simulink model "TCM_controls"  (Simulink 8.1)
settings: Solver=ode45  StartTime=0.0  StopTime=10.0  RelTol=1e-3
undefined symbols (not defined in the file): bias, sgn, sigbuilder_block, sldvsubsys, StatesInp
libraries: simulink x4, sldvlib x1
(part 1 of 2)
settings Model: Creator=mddavies  LastModifiedBy=mddavies
settings DataIOCC: SignalLoggingSaveFormat=Dataset
settings OptimizationCC: ExpressionDepthLimit=128
settings DebuggingCC: FcnCallInpInsideContextMsg=EnableAllAsError
settings GRTTargetCC: CombineOutputUpdateFcns=on  GRTInterface=off

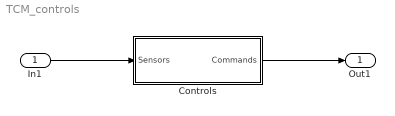
== system TCM_controls ==
  In1 : Inport
  Controls : Subsystem  RequirementInfo={} %GIDa_bfda8087_8264_4058_aa1c_dac31995074c
  Out1 : Outport
  wires:
  Controls/1(Commands) -> Out1/1
  In1/1 -> Controls/1(Sensors)

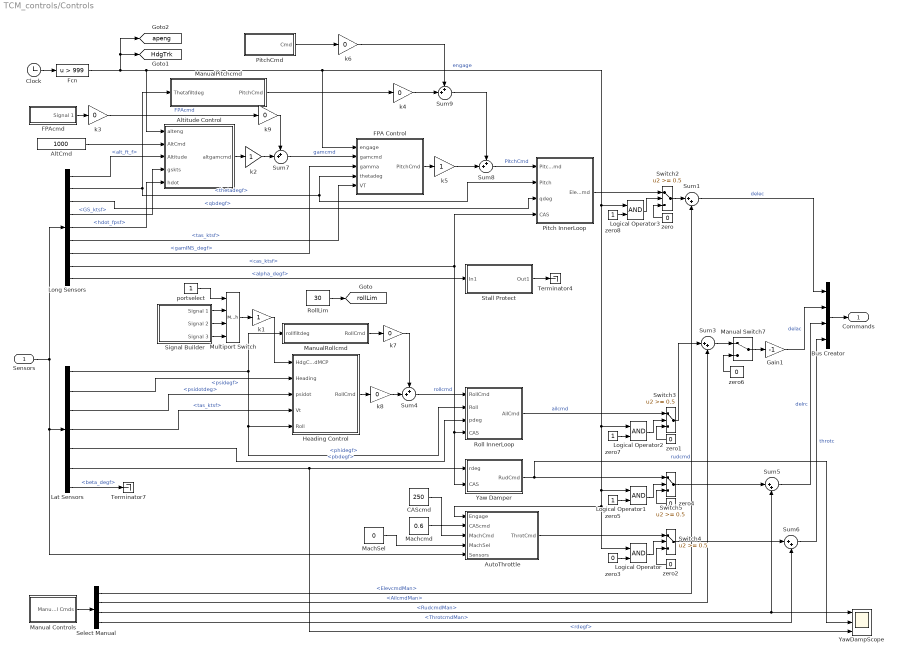
== system TCM_controls/Controls ==
  Sensors : Inport  RequirementInfo={} %GIDa_70f77869_2cec_4ef4_8031_6b1ced368b4e
  AltCmd : Constant  RequirementInfo={} %GIDa_dec5e6b5_3f45_4fcc_9d07_233f77b9af99  Value=1000
  Altitude Control : Subsystem  RequirementInfo={'other' '..\..\tcm_requirements.docx' '@Simulink_requirement_item_14' 'true' 'Altitude Control' '' } %GIDa_c6f0573f_5709_411f_9273_5bd8edb6dccb
  AutoThrottle : Subsystem  RequirementInfo={'other' '..\..\tcm_requirements.docx' '@Simulink_requirement_item_20' 'true' 'Auto Throttle' '' } %GIDa_acd8b2ec_afb4_4e6d_93a7_fadc15d05afd
  Bus Creator : BusCreator  RequirementInfo={} %GIDa_98b05b2e_4f50_4eac_8142_7ba35f876d49
  CAScmd : Constant  RequirementInfo={} %GIDa_a292a332_f5c6_4f14_a0b0_05556e3e387a  Value=250
  Clock : Clock
      settings: RequirementInfo={} %GIDa_53558b21_c326_4915_aa80_3e38ab183ff3
  FPA Control : Subsystem  RequirementInfo={'other' '..\..\tcm_requirements.docx' '@Simulink_requirement_item_15' 'true' 'FPA Control' '' } %GIDa_dac5565b_9328_42f5_a37f_49e511e4f966
  FPAcmd : Subsystem  Tag=STV Subsys  RequirementInfo={} %GIDa_1bafd98b_d710_4002_989e_dd755c1a6c5b  LoadFcn=sigbuilder_block('load');  StartFcn=sigbuilder_block('start');  StopFcn=sigbuilder_block('stop');  ClipboardFcn=sigbuilder_block('clipboard');  mask(Sigbuilder block){}
      mask help: Sigbuilder GUI
      mask init:
      | if ~strcmp(get_param(bdroot(gcbh),'SimulationStatus'),'stopped') tuvar = sigbuilder_block('maskInit'); end
      settings: CopyFcn=sigbuilder_block('copy');  DeleteFcn=sigbuilder_block('delete');  ModelCloseFcn=sigbuilder_block('modelClose');  PreSaveFcn=sigbuilder_block('preSave');  PauseFcn=sigbuilder_block('pause')  ContinueFcn=sigbuilder_block('continue')  NameChangeFcn=sigbuilder_block('namechange');  OpenFcn=sigbuilder_block('open',[437.6 199.2 550.4 400 ]);  CloseFcn=sigbuilder_block('close');
      mask Display: plot(0,0,100,100,[10,10,40,40,10],[80,20,20,80,80],[40,10],[50,50], [40,27,10],[65,72,56],[40,25,25,10],[28,28,43,43]);
  Fcn : Fcn  RequirementInfo={} %GIDa_18158dea_7053_4aed_9677_b2431daf36da  Expr=u > 999
  Gain1 : Gain  RequirementInfo={} %GIDa_de67ea91_cef0_4311_be02_dc516f1dcbf6  Gain=-1  SaturateOnIntegerOverflow=on  OutDataTypeStr=Inherit: Same as input  ParamDataTypeStr=Inherit: Same as input
  Heading Control : Subsystem  RequirementInfo={'other' '..\..\tcm_requirements.docx' '@Simulink_requirement_item_16' 'true' 'Heading Control' '' } %GIDa_4d0d22af_8d69_4b73_8cc8_bf810aba30d0
  Lat Sensors : BusSelector  RequirementInfo={} %GIDa_bff82875_4bac_4e5e_ab39_128c86e45cef  OutputSignals=phidegf,psidegf,EulerRates.psidotdeg,tas_ktsf,pbdegf,rdegf,beta_degf
  Logical Operator : Logic  RequirementInfo={} %GIDa_c9271ae6_5d7e_4e57_a9b4_c4e93f533c75  AllPortsSameDT=off  OutDataTypeStr=boolean
  Logical Operator1 : Logic  RequirementInfo={} %GIDa_bf47c128_6073_4620_9be0_bb5310186e50  AllPortsSameDT=off  OutDataTypeStr=boolean
  Logical Operator2 : Logic  RequirementInfo={} %GIDa_16878af7_9208_4803_a632_79b1d2b562ea  AllPortsSameDT=off  OutDataTypeStr=boolean
  Logical Operator3 : Logic  RequirementInfo={} %GIDa_ac9639de_92a9_41be_9497_96302f0b2ccb  AllPortsSameDT=off  OutDataTypeStr=boolean
  Long Sensors : BusSelector  RequirementInfo={} %GIDa_05f26765_1655_42bc_bb4b_9210360e7e03  OutputSignals=alt_ft_f,thetadegf,qbdegf,GS_ktsf,hdot_fpsf,tas_ktsf,gamINS_degf,cas_ktsf,alpha_degf
  MachSel : Constant  RequirementInfo={} %GIDa_406d0f5f_5220_4552_95b2_2b4717a09293  Value=0
  Machcmd : Constant  RequirementInfo={} %GIDa_bb2c15e6_ad11_44f7_ab52_0e2f70039c12  Value=0.6
  Manual Controls : Subsystem  RequirementInfo={} %GIDa_f3a5a448_da82_4163_b7bb_5bb62cb3bee1
  Manual Switch7 : ManualSwitch  RequirementInfo={} %GIDa_238d4b35_b042_4032_9af2_039cd16e9328
  ManualPitchcmd : Subsystem  RequirementInfo={} %GIDa_6f844cf0_ae74_4e05_a5ad_b4b8e37a6781
  ManualRollcmd : Subsystem  RequirementInfo={} %GIDa_c6f4980f_561d_4e8c_856f_74806f1ad0aa
  Multiport Switch : MultiPortSwitch  RequirementInfo={} %GIDa_7f9fa05b_ab44_4b7a_9c8e_e05a1b0a73ae
  Pitch InnerLoop : Subsystem  RequirementInfo={'other' '..\..\tcm_requirements.docx' '@Simulink_requirement_item_17' 'true' 'Pitch InnerLoop' '' } %GIDa_4ed92d47_0400_4ecc_8db1_4e64c2e8d840
  PitchCmd : Subsystem  RequirementInfo={} %GIDa_d85db5dc_c2d2_453e_abb8_0bd5f726e4bb
  Roll InnerLoop : Subsystem  RequirementInfo={'other' '..\..\tcm_requirements.docx' '@Simulink_requirement_item_18' 'true' 'Roll InnerLoop' '' } %GIDa_823e046a_cfe1_4d55_9112_ea4cd7fe46ad
  RollLim : Constant  RequirementInfo={} %GIDa_230728ed_bde8_446c_b764_b18561e20cc4  Value=30
  Select Manual : BusSelector  RequirementInfo={} %GIDa_92fe7b47_3580_4d0c_9647_4bc53b6f9b8a  OutputSignals=ElevcmdMan,AilcmdMan,RudcmdMan,ThrotcmdMan
  Signal Builder : Subsystem  Tag=STV Subsys  RequirementInfo={} %GIDa_de104f81_7e09_48dc_b266_08630f3c268d  LoadFcn=sigbuilder_block('load');  StartFcn=sigbuilder_block('start');  StopFcn=sigbuilder_block('stop');  ClipboardFcn=sigbuilder_block('clipboard');  mask(Sigbuilder block){}
      mask help: Sigbuilder GUI
      mask init:
      | if ~strcmp(get_param(bdroot(gcbh),'SimulationStatus'),'stopped') tuvar = sigbuilder_block('maskInit'); end
      settings: CopyFcn=sigbuilder_block('copy');  DeleteFcn=sigbuilder_block('delete');  ModelCloseFcn=sigbuilder_block('modelClose');  PreSaveFcn=sigbuilder_block('preSave');  PauseFcn=sigbuilder_block('pause')  ContinueFcn=sigbuilder_block('continue')  NameChangeFcn=sigbuilder_block('namechange');  OpenFcn=sigbuilder_block('open',[436.656 200.842 549.567 399.685 ]);  CloseFcn=sigbuilder_block('close');
      mask Display: plot(0,0,100,100,[10,10,40,40,10],[80,20,20,80,80],[40,10],[50,50], [40,27,10],[65,72,56],[40,25,25,10],[28,28,43,43]);
  Stall Protect : Subsystem  RequirementInfo={} %GIDa_81308623_113c_47aa_8ecf_809416eeaa1d
  Sum1 : Sum  RequirementInfo={} %GIDa_93388a83_d69c_4626_a784_0212b19640c2  Inputs=|++
  Sum3 : Sum  RequirementInfo={} %GIDa_5b146ea8_0844_4ecc_b2ed_46e902b595f5  Inputs=|++
  Sum4 : Sum  RequirementInfo={} %GIDa_f08d028e_f47a_4873_80ef_83f18a12d8bd  Inputs=++|
  Sum5 : Sum  RequirementInfo={} %GIDa_31e1df87_937a_4eae_9557_7a21f34925e9  Inputs=|++
  Sum6 : Sum  RequirementInfo={} %GIDa_d2e78c48_42e1_4808_ae96_99a07762e7f0  Inputs=|++
  Sum7 : Sum  RequirementInfo={} %GIDa_e99670bf_988f_4456_ae22_5591ba30988f  Inputs=++|
  Sum8 : Sum  RequirementInfo={} %GIDa_3a0866c5_ad06_43cb_b2cc_1f5b5b613d25  Inputs=++|
  Sum9 : Sum  RequirementInfo={} %GIDa_154a2fe3_c154_42b0_99bf_ba40407caa09  Inputs=++|
  Switch2 : Switch  RequirementInfo={} %GIDa_d498c400_8384_4eff_abe5_abc2c2cb970a  Threshold=0.5
  Switch3 : Switch  RequirementInfo={} %GIDa_3149d6ff_f1dc_4a93_8707_7aaa0bfbdbc5  Threshold=0.5
  Switch4 : Switch  RequirementInfo={} %GIDa_474c7c0a_d693_431e_8c01_caaa5ad223f0  Threshold=0.5
  Switch5 : Switch  RequirementInfo={} %GIDa_12969d2f_7aeb_457e_8b61_46499c9d1588  Threshold=0.5
  Terminator4 : Terminator
      settings: RequirementInfo={} %GIDa_d981aeba_8485_4cf6_9549_0eb875528307
  Terminator7 : Terminator
      settings: RequirementInfo={} %GIDa_903322f5_1a87_4f88_820f_b96602a5e0f1
  Yaw Damper : Subsystem  RequirementInfo={'other' '..\..\tcm_requirements.docx' '@Simulink_requirement_item_19' 'true' 'Yaw Damper' '' } %GIDa_e03d9e3b_12d1_4127_985c_f09d6aa1a0d4
  YawDampScope : Scope  NumInputPorts=3
      settings: RequirementInfo={} %GIDa_6e94e61d_629b_4b33_92c3_ceaeeee69283  YMin=-5~-5~-5  YMax=5~5~5  SaveName=ScopeData4
  k1 : Gain  RequirementInfo={} %GIDa_b8ae6e56_e541_4fc9_8c33_5b640a1878bf
  k2 : Gain  RequirementInfo={} %GIDa_6764272f_c68a_4a56_bdfa_0b378ddcd164
  k3 : Gain  RequirementInfo={} %GIDa_36ed0483_434a_4689_a994_f7e4d4d3ba8b  Gain=0
  k4 : Gain  RequirementInfo={} %GIDa_b90d9015_94ab_49f8_a57e_54f0da0033c5  Gain=0
  k5 : Gain  RequirementInfo={} %GIDa_6d0bd2a3_b291_46d0_acba_fbe7503f71f4
  k6 : Gain  RequirementInfo={} %GIDa_6ec47e81_80e4_46c7_bb08_7322656805f5  Gain=0
  k7 : Gain  RequirementInfo={} %GIDa_df4ad79b_1a76_4940_a29a_64f1606d84a6  Gain=0
  k8 : Gain  RequirementInfo={} %GIDa_1da1ea53_366f_4084_b3ea_cbc5e4466241  Gain=0
  k9 : Gain  RequirementInfo={} %GIDa_927c2f41_014f_4868_b1e4_5880ae857acb  Gain=0
  portselect : Constant  RequirementInfo={} %GIDa_8a2376e2_46a6_49b2_81f8_f473a2c2615b
  zero : Constant  RequirementInfo={} %GIDa_8a55f2a8_d8df_42ae_895a_6e79a0ece0e3  Value=0
  zero1 : Constant  RequirementInfo={} %GIDa_c41a1b2d_1ac1_4b5c_8545_bea2e4ad18df  Value=0
  zero2 : Constant  RequirementInfo={} %GIDa_ba22c0b1_8245_4fd4_a8d4_a7971c18af40  Value=0
  zero3 : Constant  RequirementInfo={} %GIDa_f2feaf15_c205_4351_8c8b_f665221607f7  Value=0
  zero4 : Constant  RequirementInfo={} %GIDa_7305b391_df8e_4170_9236_a6d6d9a3b599  Value=0
  zero5 : Constant  RequirementInfo={} %GIDa_c492baed_9fe4_4b04_ac61_664bb274daf7
  zero6 : Constant  RequirementInfo={} %GIDa_337c7813_2094_4eef_ae7b_8f96373121b3  Value=0
  zero7 : Constant  RequirementInfo={} %GIDa_6f701eca_c5af_4506_bbf1_05e4ee92343b
  zero8 : Constant  RequirementInfo={} %GIDa_681bde8a_1fca_46f3_8a9f_42ee6d0a1930
  Commands : Outport  RequirementInfo={} %GIDa_935988b2_9427_4adc_b718_1a527609e997
  tag scope: HdgTrk=global, apeng=global, rollLim=global
  wires:
  Lat Sensors/6 -> YawDampScope/3, Yaw Damper/1(rdeg)  "<rdegf>"
  Lat Sensors/5 -> Roll InnerLoop/3(pdeg)  "<pbdegf>"
  Lat Sensors/4 -> Heading Control/4(Vt)  "<tas_ktsf>"
  Lat Sensors/3 -> Heading Control/3(psidot)  "<psidotdeg>"
  Lat Sensors/2 -> Heading Control/2(Heading)  "<psidegf>"
  Lat Sensors/1 -> Heading Control/5(Roll), Roll InnerLoop/2(Roll), ManualRollcmd/1(rollfiltdeg)  "<phidegf>"
  AutoThrottle/1(ThrotCmd) -> Switch4/1
  Sum6/1 -> Bus Creator/4  "throtc"
  Sum5/1 -> Bus Creator/3  "delrc"
  Gain1/1 -> Bus Creator/2  "delac"
  Sum1/1 -> Bus Creator/1  "delec"
  Bus Creator/1 -> Commands/1
  Manual Switch7/1 -> Gain1/1
  k9/1 -> Sum7/1
  k3/1 -> k9/1  "FPAcmd"
  k2/1 -> Sum7/2
  Sensors/1 -> Long Sensors/1, Lat Sensors/1, AutoThrottle/5(Sensors)
  Long Sensors/1 -> Altitude Control/3(Altitude)  "<alt_ft_f>"
  Long Sensors/2 -> Pitch InnerLoop/2(Pitch), FPA Control/4(thetadeg), ManualPitchcmd/1(Thetafiltdeg)  "<thetadegf>"
  Long Sensors/8 -> Roll InnerLoop/4(CAS), Yaw Damper/2(CAS), Pitch InnerLoop/4(CAS)  "<cas_ktsf>"
  Long Sensors/7 -> FPA Control/3(gamma)  "<gamINS_degf>"
  Long Sensors/9 -> Stall Protect/1(In1)  "<alpha_degf>"
  Clock/1 -> Fcn/1
  Manual Controls/1(Manual Cmds) -> Select Manual/1
  Select Manual/1 -> Sum1/2  "<ElevcmdMan>"
  Lat Sensors/7 -> Terminator7/1  "<beta_degf>"
  Sum3/1 -> Manual Switch7/1
  Select Manual/2 -> Sum3/2  "<AilcmdMan>"
  Switch3/1 -> Sum3/1
  Sum4/1 -> Roll InnerLoop/1(RollCmd)  "rollcmd"
  Switch5/1 -> Sum5/1
  Select Manual/3 -> Sum5/2, YawDampScope/1  "<RudcmdMan>"
  CAScmd/1 -> AutoThrottle/2(CAScmd)
  Switch4/1 -> Sum6/1
  Select Manual/4 -> Sum6/2  "<ThrotcmdMan>"
  AltCmd/1 -> Altitude Control/2(AltCmd)
  k8/1 -> Sum4/2
  zero6/1 -> Manual Switch7/2
  ManualRollcmd/1(RollCmd) -> k7/1
  Switch2/1 -> Sum1/1
  zero/1 -> Switch2/3
  Fcn/1 -> Altitude Control/1(alteng), FPA Control/1(engage), Logical Operator3/1, Logical Operator2/1, Logical Operator1/1, Logical Operator/1, AutoThrottle/1(Engage), [apeng], [HdgTrk]  "engage"
  Pitch InnerLoop/1(ElevCmd) -> Switch2/1
  Altitude Control/1(altgamcmd) -> k2/1
  Sum8/1 -> Pitch InnerLoop/1(PitchCmd)  "PitchCmd"
  ManualPitchcmd/1(PitchCmd) -> k4/1
  k5/1 -> Sum8/2
  FPA Control/1(PitchCmd) -> k5/1
  Long Sensors/5 -> Altitude Control/5(hdot)  "<hdot_fpsf>"
  Sum7/1 -> FPA Control/2(gamcmd)  "gamcmd"
  Heading Control/1(RollCmd) -> k8/1
  zero1/1 -> Switch3/3
  Roll InnerLoop/1(AilCmd) -> Switch3/1  "ailcmd"
  Logical Operator/1 -> Switch4/2
  zero3/1 -> Logical Operator/2
  zero4/1 -> Switch5/3
  Logical Operator1/1 -> Switch5/2
  zero5/1 -> Logical Operator1/2
  Yaw Damper/1(RudCmd) -> Switch5/1, YawDampScope/2  "rudcmd"
  zero7/1 -> Logical Operator2/2
  Logical Operator2/1 -> Switch3/2
  zero8/1 -> Logical Operator3/2
  Logical Operator3/1 -> Switch2/2
  FPAcmd/1(Signal 1) -> k3/1
  k7/1 -> Sum4/1
  portselect/1 -> Multiport Switch/1
  Signal Builder/1(Signal 1) -> Multiport Switch/2
  Signal Builder/2(Signal 2) -> Multiport Switch/3
  Signal Builder/3(Signal 3) -> Multiport Switch/4
  Multiport Switch/1 -> k1/1
  RollLim/1 -> [rollLim]
  k1/1 -> Heading Control/1(HdgCmdMCP)
  Stall Protect/1(Out1) -> Terminator4/1
  k4/1 -> Sum9/2
  PitchCmd/1(Cmd) -> k6/1
  Sum9/1 -> Sum8/1
  k6/1 -> Sum9/1
  Long Sensors/3 -> Pitch InnerLoop/3(qdeg)  "<qbdegf>"
  Long Sensors/4 -> Altitude Control/4(gskts)  "<GS_ktsf>"
  Long Sensors/6 -> FPA Control/5(VT)  "<tas_ktsf>"
  Machcmd/1 -> AutoThrottle/3(MachCmd)
  MachSel/1 -> AutoThrottle/4(MachSel)
  zero2/1 -> Switch4/3

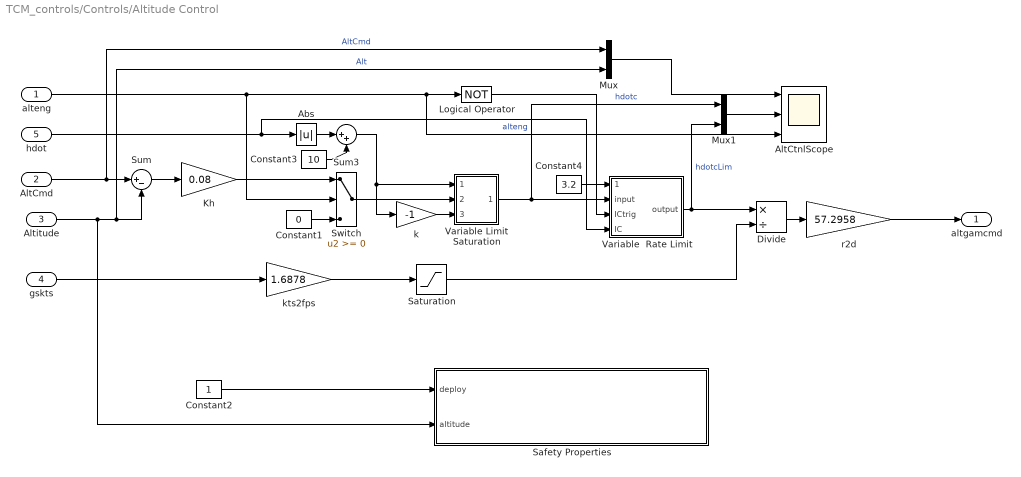
== system TCM_controls/Controls/Altitude Control ==
  alteng : Inport  RequirementInfo={} %GIDa_02633e80_0791_4996_845b_8463c8d13bdc
  AltCmd : Inport  RequirementInfo={} %GIDa_f01a5c64_5048_4ead_817f_1150ce5bafcd  Port=2
  Altitude : Inport  RequirementInfo={} %GIDa_53c75335_2a6f_43ef_8904_84222eeb9f50  Port=3
  gskts : Inport  RequirementInfo={} %GIDa_c10c2a4f_902c_4e8b_96b8_b4689bb09c59  Port=4
  hdot : Inport  RequirementInfo={} %GIDa_f0efc3ce_aa23_4913_b248_8bb3483f1443  Port=5
  Abs : Abs  RequirementInfo={} %GIDa_584ef2d4_6be5_48a2_82b7_54540d88e5ea  SaturateOnIntegerOverflow=on
  AltCtnlScope : Scope  NumInputPorts=3
      settings: RequirementInfo={} %GIDa_d2af245a_14d1_44a1_b76f_5993cea8ac6e  TimeRange=30  YMin=10000~-5~0  YMax=10200~15~1  SaveName=ScopeData3
  Constant1 : Constant  RequirementInfo={} %GIDa_142be318_071c_4741_b70e_6146455c6752  Value=0
  Constant2 : Constant  RequirementInfo={} %GIDa_aee2841a_d62a_4778_8195_69efdbd9f66c
  Constant3 : Constant  RequirementInfo={} %GIDa_4fd9daa6_86dd_480b_9e87_d7cd7d3e5ab7  Value=10
  Constant4 : Constant  RequirementInfo={} %GIDa_7712bef4_2805_4e51_9a6e_1aedf3857e74  Value=3.2
  Divide : Product  RequirementInfo={} %GIDa_518615b6_8a21_4c19_89cc_0075a8168445  Inputs=*/
  Kh : Gain  RequirementInfo={} %GIDa_2ef3e796_3e8a_4861_921e_724dc1fdaaf3  Gain=0.08
  Logical Operator : Logic  RequirementInfo={} %GIDa_dfcb40e8_cce6_4bbe_8389_8e071fcd808f  Operator=NOT
  Mux : Mux  RequirementInfo={} %GIDa_4ebb49f9_be23_440d_8228_36b8343cd879  Inputs=2
  Mux1 : Mux  RequirementInfo={} %GIDa_24366faa_de64_4cd5_a201_bde413c56619  Inputs=2
  Safety Properties : Subsystem  Tag=VerificationSubsystem  RequirementInfo={} %GIDa_fe9274ab_2722_4454_bf71_2814ec7d0b9e  DisableCoverage=on  LoadFcn=sldvsubsys('check')  TreatAsAtomicUnit=on  SimViewingDevice=on  mask(VerificationSubsystem){}
      mask init:
      | sldvsubsys('maskInit');
      settings: CopyFcn=sldvsubsys('copy');  OpenFcn=open_system(gcb,'force');
      settings: PreSaveFcn=|
      | set_param(gcb,'SimViewingDevice','on');
      | sldvsubsys('check');
      mask Help: helpview(fullfile(docroot,'toolbox','sldv','sldv.map'),'verificationsubsystem')
      mask Display: image(imread('sldvicon_versubsys.png','BackGroundColor',[1 1 1]),'center');
  Saturation : Saturate  RequirementInfo={} %GIDa_286fe06e_20c7_4df1_a50b_74f682ccfd1b  UpperLimit=1000  LowerLimit=0.0001
  Sum : Sum  RequirementInfo={} %GIDa_6fe83580_1e8a_49e8_b370_a5304e817a17  Inputs=|+-
  Sum3 : Sum  RequirementInfo={} %GIDa_2bc31f57_20de_45df_96a4_7a5cdc2ac6df  Inputs=|++  SaturateOnIntegerOverflow=on  InputSameDT=on  OutDataTypeStr=Inherit: Same as first input
  Switch : Switch  RequirementInfo={} %GIDa_d475166c_c2c0_4927_9fa4_f3e5ea7f613c
  Variable  Rate Limit : Subsystem  RequirementInfo={} %GIDa_e32f4459_34b6_4548_91a5_a7d4babef003
  Variable Limit Saturation : Subsystem  RequirementInfo={} %GIDa_15178d5d_84e2_4ba5_8f7e_4b2d48b0fa42
  k : Gain  RequirementInfo={} %GIDa_fef99285_5710_42fb_a83f_a209dfb615da  Gain=-1
  kts2fps : Gain  RequirementInfo={} %GIDa_ea7b234f_3d40_4e67_9a2d_14996b1d35d3  Gain=1.6878
  r2d : Gain  RequirementInfo={} %GIDa_7936e5b9_2b56_40ef_b6e3_68e6a59e37bd  Gain=57.2958
  altgamcmd : Outport  RequirementInfo={} %GIDa_75dd3768_76b3_4bf1_aedb_56b7c675b7de
  wires:
  Sum/1 -> Kh/1
  AltCmd/1 -> Sum/1, Mux/1  "AltCmd"
  Altitude/1 -> Safety Properties/2(altitude), Sum/2, Mux/2  "Alt"
  hdot/1 -> Abs/1, Variable  Rate Limit/4(IC)
  Abs/1 -> Sum3/1
  Constant3/1 -> Sum3/2
  k/1 -> Variable Limit Saturation/3(Lo_lim)
  Sum3/1 -> k/1, Variable Limit Saturation/1(up_lim)
  alteng/1 -> Switch/2, Logical Operator/1, AltCtnlScope/3  "alteng"
  gskts/1 -> kts2fps/1
  Divide/1 -> r2d/1
  r2d/1 -> altgamcmd/1
  Logical Operator/1 -> Variable  Rate Limit/3(ICtrig)
  Variable Limit Saturation/1(Out1) -> Variable  Rate Limit/2(input), Mux1/1  "hdotc"
  Constant4/1 -> Variable  Rate Limit/1(ratelim)
  Variable  Rate Limit/1(output) -> Divide/1, Mux1/2  "hdotcLim"
  kts2fps/1 -> Saturation/1
  Saturation/1 -> Divide/2
  Switch/1 -> Variable Limit Saturation/2(SigIn)
  Kh/1 -> Switch/1
  Constant1/1 -> Switch/3
  Mux/1 -> AltCtnlScope/1
  Mux1/1 -> AltCtnlScope/2
  Constant2/1 -> Safety Properties/1(deploy)

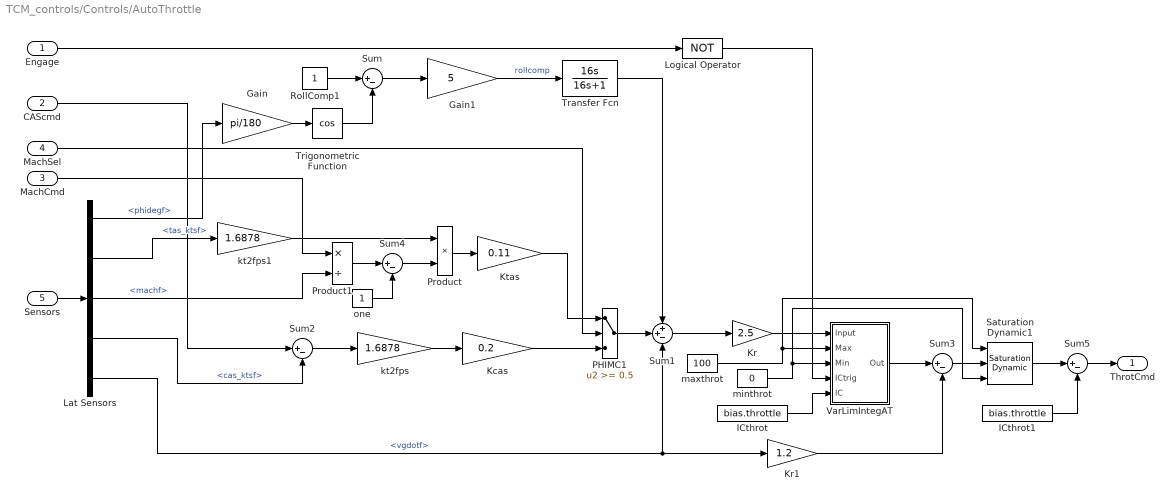
== system TCM_controls/Controls/AutoThrottle ==
  Engage : Inport  RequirementInfo={} %GIDa_c78350fb_fa81_4a6c_8041_709e76a511d5
  CAScmd : Inport  RequirementInfo={} %GIDa_d62d65f5_bfde_45ec_b3c2_4a1562c916d6  Port=2
  MachCmd : Inport  RequirementInfo={} %GIDa_6e18ebad_ed77_45d2_aa73_dcf4bccb826c  Port=3
  MachSel : Inport  RequirementInfo={} %GIDa_e1e0a91a_092e_4073_8070_c3a59f5b97f0  Port=4
  Sensors : Inport  RequirementInfo={} %GIDa_04629c4c_6ba1_49d3_8fc4_922875642bf0  Port=5
  Gain : Gain  RequirementInfo={} %GIDa_f72af6a8_661d_4465_a155_21ee211addf4  Gain=pi/180
  Gain1 : Gain  RequirementInfo={} %GIDa_d1c1e1b8_ce39_46fd_8f6a_f7539e22cf0a  Gain=5
  ICthrot : Constant  RequirementInfo={} %GIDa_2fcdee91_9306_45f9_9b2a_322564fd6a9a  Value=bias.throttle  SampleTime=-1
  ICthrot1 : Constant  RequirementInfo={} %GIDa_e3cb9808_12a0_449b_a4a7_26c21a0dd8b2  Value=bias.throttle  SampleTime=-1
  Kcas : Gain  RequirementInfo={} %GIDa_ac1acf1d_597b_4e61_a972_9454b39e0927  Gain=0.2
  Kr : Gain  RequirementInfo={} %GIDa_db49a02a_6b80_49c5_91c0_1fbc690ab318  Gain=2.5
  Kr1 : Gain  RequirementInfo={} %GIDa_73ff3e33_02cb_4dbd_abf2_ecfbb60a33a4  Gain=1.2
  Ktas : Gain  RequirementInfo={} %GIDa_3937ba58_9f30_4ce2_9403_44b9fbdbbcdb  Gain=0.11
  Lat Sensors : BusSelector  RequirementInfo={} %GIDa_d4684bc5_15b9_4aca_86c1_b91af86b245e  OutputSignals=phidegf,tas_ktsf,machf,cas_ktsf,vgdotf
  Logical Operator : Logic  RequirementInfo={} %GIDa_4512f38f_f881_42c2_9fc9_d7785cd1fe48  Operator=NOT  AllPortsSameDT=off  OutDataTypeStr=boolean
  PHIMC1 : Switch  RequirementInfo={} %GIDa_38937a7f_5f70_4f47_9d3f_4f45007894cb  Threshold=0.5  SampleTime=0.02  SaturateOnIntegerOverflow=on
  Product : Product  RequirementInfo={} %GIDa_9d6aee68_f232_4ee5_a7bb_5058db639735  RndMeth=Zero
  Product1 : Product  RequirementInfo={} %GIDa_9bd25c5e_ccc8_467b_beb1_404913d69c67  Inputs=*/  RndMeth=Zero
  RollComp1 : Constant  RequirementInfo={} %GIDa_6f64c878_e625_47af_bbbc_1f46b151678b  SampleTime=-1
  Saturation Dynamic1 : simulink/Discontinuities/Saturation Dynamic  RequirementInfo={} %GIDa_9fa3fc13_ab06_443e_852f_62ed3f5eb5ad  OutMin=[]  OutMax=[]  OutDataTypeStr=Inherit: Same as second input  OutDataType=sfix(16)  OutScaling=2^-10  DoSatur=off
  Sum : Sum  RequirementInfo={} %GIDa_c96b5531_0d8e_4ce9_972a_a12a3c140a36  Inputs=|+-
  Sum1 : Sum  RequirementInfo={} %GIDa_ff122384_47e7_4541_b600_e49509ecbdcb  Inputs=++-
  Sum2 : Sum  RequirementInfo={} %GIDa_2a4657ac_602b_42c1_9aef_62135f38a158  Inputs=|+-
  Sum3 : Sum  RequirementInfo={} %GIDa_b04521ce_5b21_43fe_adca_81cc300ef696  Inputs=|+-
  Sum4 : Sum  RequirementInfo={} %GIDa_66decbf6_63a3_4144_8b9d_0f9ac1e88bb6  Inputs=|+-
  Sum5 : Sum  RequirementInfo={} %GIDa_00c82fc8_7d29_4e94_bb47_a680e8082b0d  Inputs=|+-
  Transfer Fcn : TransferFcn  RequirementInfo={} %GIDa_8a88fa97_6339_4910_8a70_ee6567c6dac7  Numerator=[16 0]  Denominator=[16 1]
  Trigonometric Function : Trigonometry  RequirementInfo={} %GIDa_e383f247_a1b6_4070_acb4_f0617f4ed0f0  Operator=cos
  VarLimIntegAT : Subsystem  RequirementInfo={} %GIDa_f396fc90_a185_45e5_987a_0bb57ea297cb
  kt2fps : Gain  RequirementInfo={} %GIDa_1fc554ce_56ee_47bc_880a_0cca1ceec330  Gain=1.6878
  kt2fps1 : Gain  RequirementInfo={} %GIDa_7ac87cf0_6bf6_4d0a_a4bc_65e2bc24c465  Gain=1.6878
  maxthrot : Constant  RequirementInfo={} %GIDa_9fb28dbc_f107_4823_9058_9630c9255e8b  Value=100  SampleTime=-1
  minthrot : Constant  RequirementInfo={} %GIDa_c621bed3_d7f5_471f_a710_16dd9df2d68f  Value=0  SampleTime=-1
  one : Constant  RequirementInfo={} %GIDa_cd20c5fe_ca4b_4fec_b358_54a99c4323c8  SampleTime=-1
  ThrotCmd : Outport  RequirementInfo={} %GIDa_da1d0932_be70_457f_b044_35341889dcb0
  wires:
  CAScmd/1 -> Sum2/1
  Sum2/1 -> kt2fps/1
  Sum1/1 -> Kr/1
  kt2fps/1 -> Kcas/1
  Kr/1 -> VarLimIntegAT/1(Input)
  Lat Sensors/5 -> Sum1/3, Kr1/1  "<vgdotf>"
  Kr1/1 -> Sum3/2
  Gain1/1 -> Transfer Fcn/1  "rollcomp"
  Sum/1 -> Gain1/1
  Trigonometric Function/1 -> Sum/2
  RollComp1/1 -> Sum/1
  Gain/1 -> Trigonometric Function/1
  Product1/1 -> Sum4/1
  one/1 -> Sum4/2
  Sum4/1 -> Product/2
  kt2fps1/1 -> Product/1
  Product/1 -> Ktas/1
  ICthrot/1 -> VarLimIntegAT/5(IC)
  Sum5/1 -> ThrotCmd/1
  ICthrot1/1 -> Sum5/2
  maxthrot/1 -> VarLimIntegAT/2(Max), Saturation Dynamic1/1
  minthrot/1 -> VarLimIntegAT/3(Min), Saturation Dynamic1/3
  VarLimIntegAT/1(Out) -> Sum3/1
  Sum3/1 -> Saturation Dynamic1/2
  Saturation Dynamic1/1 -> Sum5/1
  PHIMC1/1 -> Sum1/2
  Kcas/1 -> PHIMC1/3
  Ktas/1 -> PHIMC1/1
  Transfer Fcn/1 -> Sum1/1
  Sensors/1 -> Lat Sensors/1
  Lat Sensors/1 -> Gain/1  "<phidegf>"
  Lat Sensors/2 -> kt2fps1/1  "<tas_ktsf>"
  Lat Sensors/4 -> Sum2/2  "<cas_ktsf>"
  Logical Operator/1 -> VarLimIntegAT/4(ICtrig)
  Engage/1 -> Logical Operator/1
  MachSel/1 -> PHIMC1/2
  MachCmd/1 -> Product1/1
  Lat Sensors/3 -> Product1/2  "<machf>"

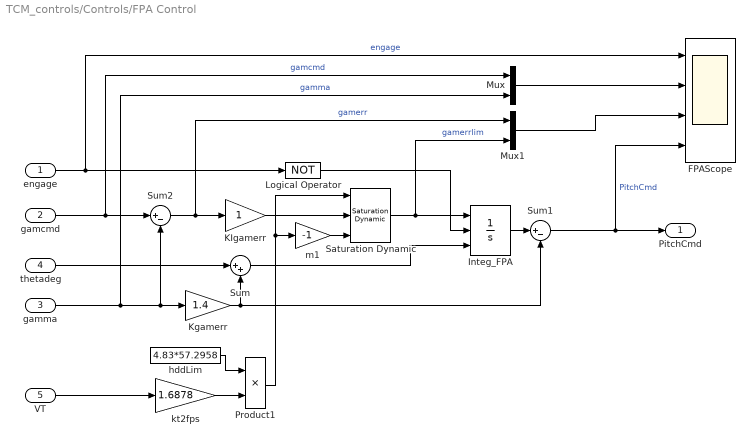
== system TCM_controls/Controls/FPA Control ==
  engage : Inport  RequirementInfo={} %GIDa_91c37145_4feb_4e56_8ba4_c1444bccd725
  gamcmd : Inport  RequirementInfo={} %GIDa_35b48e29_8b9c_4d71_bc7e_7f801982c35c  Port=2
  gamma : Inport  RequirementInfo={} %GIDa_7cbea00d_7d0f_450c_a5ed_a36a9e878ad0  Port=3
  thetadeg : Inport  RequirementInfo={} %GIDa_4586afe0_6b15_41e1_92d5_c5cb5fb147ef  Port=4
  VT : Inport  RequirementInfo={} %GIDa_6bfccaa8_1761_4626_8ec4_ffc0a99026f2  Port=5
  FPAScope : Scope  NumInputPorts=4
      settings: RequirementInfo={} %GIDa_6521d4bd_734b_43fe_9864_4305ee45935d  YMin=-1~-5~-2~-5  YMax=2~5~2~10  SaveName=ScopeData12
  Integ_FPA : Integrator  RequirementInfo={} %GIDa_4618b833_ba21_4a0d_a2fc_2134a3fdeaf2  ExternalReset=level  InitialConditionSource=external  IgnoreLimit=on
  KIgamerr : Gain  RequirementInfo={} %GIDa_e7aeae8d_827d_4b55_88b8_d1146319fac7
  Kgamerr : Gain  RequirementInfo={} %GIDa_86f0c6f9_3df3_4585_b0c9_834159dda395  Gain=1.4
  Logical Operator : Logic  RequirementInfo={} %GIDa_38a821e1_72c6_4a66_890a_b37f371667cc  Operator=NOT  AllPortsSameDT=off  OutDataTypeStr=boolean
  Mux : Mux  RequirementInfo={} %GIDa_00ae75ae_0d91_468f_8bef_95619be93ca4  Inputs=2
  Mux1 : Mux  RequirementInfo={} %GIDa_1f83504d_893a_4b09_bc5e_37512c768209  Inputs=2
  Product1 : Product  RequirementInfo={} %GIDa_6a4eb71a_e02e_42ca_b616_9047e49f49ad  RndMeth=Zero
  Saturation Dynamic : simulink/Discontinuities/Saturation Dynamic  RequirementInfo={} %GIDa_44aa7d72_cca6_47f1_9171_f5724db5be1d  OutMin=[]  OutMax=[]  OutDataTypeStr=Inherit: Same as second input  OutDataType=fixdt(1, 16)  OutScaling=2^-10  DoSatur=off
  Sum : Sum  RequirementInfo={} %GIDa_d76ccd44_16d8_45d1_a5c8_8cb855f3fa60  Inputs=|++
  Sum1 : Sum  RequirementInfo={} %GIDa_b2cc6a5b_6a0c_43d6_8e07_ed52d21ae106  Inputs=|+-
  Sum2 : Sum  RequirementInfo={} %GIDa_face43d4_08a8_46f4_83de_258637401c1a  Inputs=|+-
  hddLim : Constant  RequirementInfo={} %GIDa_33972148_d26a_40f1_920d_6c8d069e5033  Value=4.83*57.2958
  kt2fps : Gain  RequirementInfo={} %GIDa_000eb7a6_2566_45a9_a1f0_9c22b86ad75e  Gain=1.6878
  m1 : Gain  RequirementInfo={} %GIDa_5ffae559_17f0_4758_b2a4_292a59072b8b  Gain=-1
  PitchCmd : Outport  RequirementInfo={} %GIDa_d8cb079f_c0bb_4316_969b_9657e50c7147
  wires:
  Sum1/1 -> PitchCmd/1, FPAScope/4  "PitchCmd"
  Kgamerr/1 -> Sum1/2, Sum/2
  Integ_FPA/1 -> Sum1/1
  gamma/1 -> Kgamerr/1, Sum2/2, Mux/2  "gamma"
  thetadeg/1 -> Sum/1
  Sum/1 -> Integ_FPA/3
  engage/1 -> Logical Operator/1, FPAScope/1  "engage"
  Logical Operator/1 -> Integ_FPA/2
  kt2fps/1 -> Product1/2
  hddLim/1 -> Product1/1
  Product1/1 -> Saturation Dynamic/1, m1/1
  VT/1 -> kt2fps/1
  Saturation Dynamic/1 -> Integ_FPA/1, Mux1/2  "gamerrlim"
  KIgamerr/1 -> Saturation Dynamic/2
  m1/1 -> Saturation Dynamic/3
  Sum2/1 -> KIgamerr/1, Mux1/1  "gamerr"
  gamcmd/1 -> Sum2/1, Mux/1  "gamcmd"
  Mux/1 -> FPAScope/2
  Mux1/1 -> FPAScope/3

== system TCM_controls/Controls/FPAcmd ==
  Demux : Demux  Tag=STV Demux  RequirementInfo={} %GIDa_8777f547_aef8_43e3_8546_8c52671b52a1  Outputs=1
  FromWs : FromWorkspace  Tag=STV FromWs  RequirementInfo={} %GIDa_c1570c47_0b24_4554_af2f_bb2cfdd31430  VariableName=tuvar  SampleTime=0  SigBuilderData=DataTag0  VnvData=DataTag1
      SigBuilderData=|
      | common.afterFinalStr = 'Extrapolate'
      | common.sampleTime = 0
      | dataSet.timeRange = [0 10]
      | dataSet.name = 'Group 1'
      | sbobj.Groups.Name = 'Group 1'
      | sbobj.Groups.Signals.Name = 'Signal 1'
      | sbobj.Groups.Signals.XData = [0 1 1 6 10]
      | sbobj.Groups.Signals.YData = [0 0 1 1 1]
  Signal 1 : Outport  Tag=STV Outport  RequirementInfo={} %GIDa_db3906c6_a893_4994_8e4d_785984a8716e
  wires:
  Demux/1 -> Signal 1/1
  FromWs/1 -> Demux/1

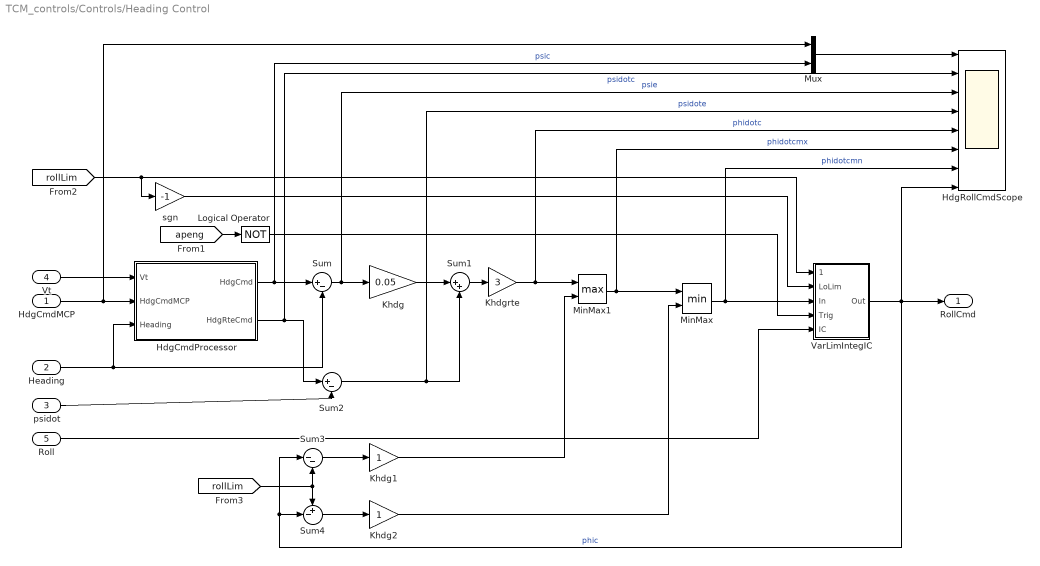
== system TCM_controls/Controls/Heading Control ==
  HdgCmdMCP : Inport  RequirementInfo={} %GIDa_5d8974ae_6a69_4daa_9dd2_fbeb998e42e6
  Heading : Inport  RequirementInfo={} %GIDa_8d3e0609_0151_4eb7_a305_e3dc039d710d  Port=2
  psidot : Inport  RequirementInfo={} %GIDa_ec8d66e0_b06b_4f2d_be9b_ad9375884a84  Port=3
  Vt : Inport  RequirementInfo={} %GIDa_ebccda4a_b5e4_4b69_a1c2_58079894eb38  Port=4
  Roll : Inport  RequirementInfo={} %GIDa_728cddf4_2276_48d9_9c20_503dc5676c7d  Port=5
  HdgCmdProcessor : Subsystem  RequirementInfo={} %GIDa_6fc1308f_5c9f_4c2b_bfe9_ed64c461b3a5
  HdgRollCmdScope : Scope  NumInputPorts=8
      settings: RequirementInfo={} %GIDa_c9e2c47d_239a_4dfb_b8c8_6440c9270e1b  YMin=-30~-30~-10~-10~-4~-10~0~-5  YMax=30~30~10~10~4~10~1~5  SaveName=ScopeData7
  Khdg : Gain  RequirementInfo={} %GIDa_67d8533f_dec2_4d31_be19_58178eb765d6  Gain=0.05
  Khdg1 : Gain  RequirementInfo={} %GIDa_c1dbdcb6_8763_4cea_b5ee_bae53f79bdf5
  Khdg2 : Gain  RequirementInfo={} %GIDa_f021ef5a_e24b_482e_9107_17b2c3567a49
  Khdgrte : Gain  RequirementInfo={} %GIDa_f33f2c16_e0d7_41ac_b62d_2b1d4399e4b7  Gain=3
  Logical Operator : Logic  RequirementInfo={} %GIDa_528db436_dd65_404c_8df3_1756247e5783  Operator=NOT  AllPortsSameDT=off  OutDataTypeStr=boolean
  MinMax : MinMax  RequirementInfo={} %GIDa_f41f95fb_6e85_41f1_a480_e253c1db82c0  Inputs=2
  MinMax1 : MinMax  RequirementInfo={} %GIDa_74f3f409_e21c_40f9_8d4c_3ba251e0e5ce  Function=max  Inputs=2
  Mux : Mux  RequirementInfo={} %GIDa_30d1c341_f001_4afd_92b4_cd5f41fb7188  Inputs=2
  Sum : Sum  RequirementInfo={} %GIDa_b0ec92c1_2f2c_49e8_89fd_309eb1585dff  Inputs=|+-
  Sum1 : Sum  RequirementInfo={} %GIDa_35e19418_3638_4783_bb09_588238e570b8  Inputs=|++
  Sum2 : Sum  RequirementInfo={} %GIDa_54390491_70db_4a32_a0d2_c12dcd7c1b72  Inputs=|+-
  Sum3 : Sum  RequirementInfo={} %GIDa_6cc3641f_51e2_4302_bb3f_ab122b5093a9  Inputs=|--
  Sum4 : Sum  RequirementInfo={} %GIDa_e3d72566_f816_4118_9f3b_7329441cd5d6  Inputs=+-|
  VarLimIntegIC : Subsystem  RequirementInfo={} %GIDa_4c9a4df1_da64_4e1f_a78c_925dc03f037b
  sgn : Gain  RequirementInfo={} %GIDa_25922014_f583_46a7_b7fc_0acec1d4d5bf  Gain=-1
  RollCmd : Outport  RequirementInfo={} %GIDa_05e65c6f_d197_4121_a41e_457039d08439
  wires:
  Heading/1 -> Sum/2, HdgCmdProcessor/3(Heading)
  HdgCmdProcessor/1(HdgCmd) -> Sum/1, Mux/2  "psic"
  Sum/1 -> Khdg/1, HdgRollCmdScope/3  "psie"
  Khdg/1 -> Sum1/1
  Sum2/1 -> Sum1/2, HdgRollCmdScope/4  "psidote"
  HdgCmdProcessor/2(HdgRteCmd) -> Sum2/1, HdgRollCmdScope/2  "psidotc"
  psidot/1 -> Sum2/2
  Vt/1 -> HdgCmdProcessor/1(Vt)
  HdgCmdMCP/1 -> HdgCmdProcessor/2(HdgCmdMCP), Mux/1
  VarLimIntegIC/1(Out) -> RollCmd/1, Sum3/1, Sum4/2, HdgRollCmdScope/8  "phic"
  [rollLim] -> VarLimIntegIC/1(UpLim), sgn/1
  sgn/1 -> VarLimIntegIC/2(LoLim)
  [rollLim] -> Sum3/2, Sum4/1
  Sum1/1 -> Khdgrte/1
  MinMax1/1 -> MinMax/1, HdgRollCmdScope/6  "phidotcmx"
  MinMax/1 -> VarLimIntegIC/3(In), HdgRollCmdScope/7  "phidotcmn"
  [apeng] -> Logical Operator/1
  Sum3/1 -> Khdg1/1
  Sum4/1 -> Khdg2/1
  Khdg1/1 -> MinMax1/2
  Khdg2/1 -> MinMax/2
  Roll/1 -> VarLimIntegIC/5(IC)
  Khdgrte/1 -> MinMax1/1, HdgRollCmdScope/5  "phidotc"
  Logical Operator/1 -> VarLimIntegIC/4(Trig)
  Mux/1 -> HdgRollCmdScope/1

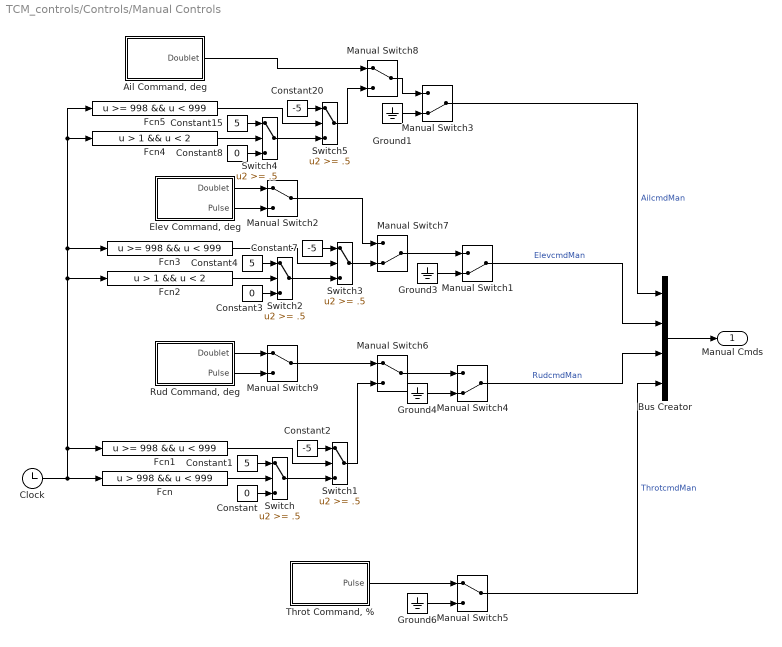
== system TCM_controls/Controls/Manual Controls ==
  "Ail Command, deg" : Subsystem  Tag=STV Subsys  RequirementInfo={} %GIDa_4587aa49_2f39_4576_83ed_6bb9d5999693  LoadFcn=sigbuilder_block('load');  StartFcn=sigbuilder_block('start');  StopFcn=sigbuilder_block('stop');  ClipboardFcn=sigbuilder_block('clipboard');  mask(Sigbuilder block){}
      mask help: Sigbuilder GUI
      mask init:
      | if ~strcmp(get_param(bdroot(gcbh),'SimulationStatus'),'stopped') tuvar = sigbuilder_block('maskInit'); end
      settings: CopyFcn=sigbuilder_block('copy');  DeleteFcn=sigbuilder_block('delete');  ModelCloseFcn=sigbuilder_block('modelClose');  PreSaveFcn=sigbuilder_block('preSave');  PauseFcn=sigbuilder_block('pause')  ContinueFcn=sigbuilder_block('continue')  NameChangeFcn=sigbuilder_block('namechange');  OpenFcn=sigbuilder_block('open',[20.16 261.12 550.08 400.32 ]);  CloseFcn=sigbuilder_block('close');
      mask Display: plot(0,0,100,100,[10,10,40,40,10],[80,20,20,80,80],[40,10],[50,50], [40,27,10],[65,72,56],[40,25,25,10],[28,28,43,43]);
  Bus Creator : BusCreator  RequirementInfo={} %GIDa_8ed9ea0a_6966_4635_8101_ebd3af6c754a
  Clock : Clock
      settings: RequirementInfo={} %GIDa_5136987a_87a9_4dea_8466_bb581d5eea61
  Constant : Constant  RequirementInfo={} %GIDa_79648cf5_d189_4f55_ab72_d926080d3eec  Value=0
  Constant1 : Constant  RequirementInfo={} %GIDa_ee59fecd_e7f7_4732_b9f9_9b0369b8ceff  Value=5
  Constant15 : Constant  RequirementInfo={} %GIDa_ae0d92fc_5d27_4f31_8942_ee64460c7fa2  Value=5
  Constant2 : Constant  RequirementInfo={} %GIDa_0d316e90_c54d_499d_9581_4117918d3145  Value=-5
  Constant20 : Constant  RequirementInfo={} %GIDa_8c43a1dd_430b_46b2_800a_154f34d73d0d  Value=-5
  Constant3 : Constant  RequirementInfo={} %GIDa_edc7ed9c_7566_4fae_90b3_6113606788ee  Value=0
  Constant4 : Constant  RequirementInfo={} %GIDa_7cad298d_1eb3_4afc_b1e3_4d516be037af  Value=5
  Constant7 : Constant  RequirementInfo={} %GIDa_74e8c061_47a3_4c5c_aa93_53dbb32a0b0f  Value=-5
  Constant8 : Constant  RequirementInfo={} %GIDa_dc1b0779_4fb1_44b9_b332_40a4bed07b31  Value=0
  "Elev Command, deg" : Subsystem  Tag=STV Subsys  RequirementInfo={} %GIDa_28e6eef5_6a32_44de_93be_2287055b4fc1  LoadFcn=sigbuilder_block('load');  StartFcn=sigbuilder_block('start');  StopFcn=sigbuilder_block('stop');  ClipboardFcn=sigbuilder_block('clipboard');  mask(Sigbuilder block){}
      mask help: Sigbuilder GUI
      mask init:
      | if ~strcmp(get_param(bdroot(gcbh),'SimulationStatus'),'stopped') tuvar = sigbuilder_block('maskInit'); end
      settings: CopyFcn=sigbuilder_block('copy');  DeleteFcn=sigbuilder_block('delete');  ModelCloseFcn=sigbuilder_block('modelClose');  PreSaveFcn=sigbuilder_block('preSave');  PauseFcn=sigbuilder_block('pause')  ContinueFcn=sigbuilder_block('continue')  NameChangeFcn=sigbuilder_block('namechange');  OpenFcn=sigbuilder_block('open',[550.08 198.72 550.08 400.32 ]);  CloseFcn=sigbuilder_block('close');
      mask Display: plot(0,0,100,100,[10,10,40,40,10],[80,20,20,80,80],[40,10],[50,50], [40,27,10],[65,72,56],[40,25,25,10],[28,28,43,43]);
  Fcn : Fcn  RequirementInfo={} %GIDa_16cb0ec0_ce51_4d62_b897_c8b23f4fae82  Expr=u > 998 && u < 999
  Fcn1 : Fcn  RequirementInfo={} %GIDa_ddd6ba77_d7dc_456e_a727_0847d9d21ec6  Expr=u >= 998 && u < 999
  Fcn2 : Fcn  RequirementInfo={} %GIDa_48172823_adcc_446c_922b_4ce405d0e000  Expr=u > 1 && u < 2
  Fcn3 : Fcn  RequirementInfo={} %GIDa_7d8ac5bc_50af_4158_97e6_fc82f388f58f  Expr=u >= 998 && u < 999
  Fcn4 : Fcn  RequirementInfo={} %GIDa_2b257206_2e2c_4c4a_9d9d_60e7f8c99ae9  Expr=u > 1 && u < 2
  Fcn5 : Fcn  RequirementInfo={} %GIDa_dd294485_666c_4fff_9ab1_36a00009b93d  Expr=u >= 998 && u < 999
  Ground1 : Ground  RequirementInfo={} %GIDa_2eb618ad_08d8_4d3f_9872_f956525370a9
  Ground3 : Ground  RequirementInfo={} %GIDa_85524bb7_1368_4292_b973_ccc838119172
  Ground4 : Ground  RequirementInfo={} %GIDa_b294035e_1a93_45cd_a422_ea80c2f613a1
  Ground6 : Ground  RequirementInfo={} %GIDa_c1db9543_8324_4cf3_95ad_70579245d872
  Manual Switch1 : ManualSwitch  RequirementInfo={} %GIDa_bd770411_5d43_4c13_8299_9a6f1597552c  CurrentSetting=0
  Manual Switch2 : ManualSwitch  RequirementInfo={} %GIDa_135c6bcf_702a_4ef5_be89_d256d8e2afdb
  Manual Switch3 : ManualSwitch  RequirementInfo={} %GIDa_556fbe42_1251_4231_a7c3_2c3283547d24  CurrentSetting=0
  Manual Switch4 : ManualSwitch  RequirementInfo={} %GIDa_725bf034_98c3_4d22_a0c2_08542f11bcf1  CurrentSetting=0
  Manual Switch5 : ManualSwitch  RequirementInfo={} %GIDa_0ea7f2e0_ba84_4c7c_bdb3_b1d68c877a6d
  Manual Switch6 : ManualSwitch  RequirementInfo={} %GIDa_56efb77a_9620_47ce_99b4_378a0f3198d8
  Manual Switch7 : ManualSwitch  RequirementInfo={} %GIDa_59450228_58ee_424c_b8c9_213e5be8e61d  CurrentSetting=0
  Manual Switch8 : ManualSwitch  RequirementInfo={} %GIDa_eeb14a55_d1b6_4e67_b573_6d3b0e40ea2a
  Manual Switch9 : ManualSwitch  RequirementInfo={} %GIDa_d1628304_2438_49e6_bec7_91f00a22f1f6
  "Rud Command, deg" : Subsystem  Tag=STV Subsys  RequirementInfo={} %GIDa_81de0af2_0acd_4536_b7be_0a351afc5b00  LoadFcn=sigbuilder_block('load');  StartFcn=sigbuilder_block('start');  StopFcn=sigbuilder_block('stop');  ClipboardFcn=sigbuilder_block('clipboard');  mask(Sigbuilder block){}
      mask help: Sigbuilder GUI
      mask init:
      | if ~strcmp(get_param(bdroot(gcbh),'SimulationStatus'),'stopped') tuvar = sigbuilder_block('maskInit'); end
      settings: CopyFcn=sigbuilder_block('copy');  DeleteFcn=sigbuilder_block('delete');  ModelCloseFcn=sigbuilder_block('modelClose');  PreSaveFcn=sigbuilder_block('preSave');  PauseFcn=sigbuilder_block('pause')  ContinueFcn=sigbuilder_block('continue')  NameChangeFcn=sigbuilder_block('namechange');  OpenFcn=sigbuilder_block('open',[437.6 199.2 550.4 400 ]);  CloseFcn=sigbuilder_block('close');
      mask Display: plot(0,0,100,100,[10,10,40,40,10],[80,20,20,80,80],[40,10],[50,50], [40,27,10],[65,72,56],[40,25,25,10],[28,28,43,43]);
  Switch : Switch  RequirementInfo={} %GIDa_e4984542_004c_4610_afdd_2525a6239768  Threshold=.5
  Switch1 : Switch  RequirementInfo={} %GIDa_1bd4af8c_8c4a_41fd_b1c4_583fa96ae51b  Threshold=.5
  Switch2 : Switch  RequirementInfo={} %GIDa_f03c5078_85e5_4a00_9ed9_7384e557dfda  Threshold=.5
  Switch3 : Switch  RequirementInfo={} %GIDa_48ee1b50_511f_4100_9a7c_099f3c47dabd  Threshold=.5
  Switch4 : Switch  RequirementInfo={} %GIDa_3c9b74e2_cb78_482e_898c_587a143aad5c  Threshold=.5
  Switch5 : Switch  RequirementInfo={} %GIDa_2a55bf23_ff25_44b2_80d4_f0c7322ba493  Threshold=.5
  "Throt Command, %" : Subsystem  Tag=STV Subsys  RequirementInfo={} %GIDa_e665f8ad_1c0a_4639_91cb_b74bed0a9f9a  LoadFcn=sigbuilder_block('load');  StartFcn=sigbuilder_block('start');  StopFcn=sigbuilder_block('stop');  ClipboardFcn=sigbuilder_block('clipboard');  mask(Sigbuilder block){}
      mask help: Sigbuilder GUI
      mask init:
      | if ~strcmp(get_param(bdroot(gcbh),'SimulationStatus'),'stopped') tuvar = sigbuilder_block('maskInit'); end
      settings: CopyFcn=sigbuilder_block('copy');  DeleteFcn=sigbuilder_block('delete');  ModelCloseFcn=sigbuilder_block('modelClose');  PreSaveFcn=sigbuilder_block('preSave');  PauseFcn=sigbuilder_block('pause')  ContinueFcn=sigbuilder_block('continue')  NameChangeFcn=sigbuilder_block('namechange');  OpenFcn=sigbuilder_block('open',[436.656 201.841 549.567 399.685 ]);  CloseFcn=sigbuilder_block('close');
      mask Display: plot(0,0,100,100,[10,10,40,40,10],[80,20,20,80,80],[40,10],[50,50], [40,27,10],[65,72,56],[40,25,25,10],[28,28,43,43]);
  Manual Cmds : Outport  RequirementInfo={} %GIDa_ba3968b0_a156_451b_a741_54db42cce3bd
  wires:
  Ground1/1 -> Manual Switch3/2
  Ground3/1 -> Manual Switch1/2
  "Elev Command, deg"/1(Doublet) -> Manual Switch2/1
  "Elev Command, deg"/2(Pulse) -> Manual Switch2/2
  Ground4/1 -> Manual Switch4/2
  Ground6/1 -> Manual Switch5/2
  "Throt Command, %"/1(Pulse) -> Manual Switch5/1
  Fcn/1 -> Switch/2
  Constant1/1 -> Switch/1
  Constant/1 -> Switch/3
  Switch/1 -> Switch1/3
  Constant2/1 -> Switch1/1
  Fcn1/1 -> Switch1/2
  Clock/1 -> Fcn/1, Fcn1/1, Fcn2/1, Fcn3/1, Fcn5/1, Fcn4/1
  Manual Switch6/1 -> Manual Switch4/1
  Switch1/1 -> Manual Switch6/2
  Fcn2/1 -> Switch2/2
  Constant4/1 -> Switch2/1
  Constant3/1 -> Switch2/3
  Switch2/1 -> Switch3/3
  Constant7/1 -> Switch3/1
  Fcn3/1 -> Switch3/2
  Manual Switch7/1 -> Manual Switch1/1
  Switch3/1 -> Manual Switch7/2
  Manual Switch2/1 -> Manual Switch7/1
  Fcn4/1 -> Switch4/2
  Constant15/1 -> Switch4/1
  Constant8/1 -> Switch4/3
  Switch4/1 -> Switch5/3
  Constant20/1 -> Switch5/1
  Fcn5/1 -> Switch5/2
  Manual Switch8/1 -> Manual Switch3/1
  Switch5/1 -> Manual Switch8/2
  "Ail Command, deg"/1(Doublet) -> Manual Switch8/1
  Manual Switch3/1 -> Bus Creator/1  "AilcmdMan"
  Manual Switch1/1 -> Bus Creator/2  "ElevcmdMan"
  Manual Switch4/1 -> Bus Creator/3  "RudcmdMan"
  Manual Switch5/1 -> Bus Creator/4  "ThrotcmdMan"
  Bus Creator/1 -> Manual Cmds/1
  "Rud Command, deg"/1(Doublet) -> Manual Switch9/1
  "Rud Command, deg"/2(Pulse) -> Manual Switch9/2
  Manual Switch9/1 -> Manual Switch6/1

== system TCM_controls/Controls/ManualPitchcmd ==
  Thetafiltdeg : Inport  RequirementInfo={} %GIDa_afb5deeb_2c85_4e1c_a12d_c21e8556e5ee
  Constant : Constant  RequirementInfo={} %GIDa_c20cd1e7_1b7f_4999_8da3_2fd71bf2b43e  Value=3
  Constant1 : Constant  RequirementInfo={} %GIDa_0a3827e2_5f77_4649_bc7d_6b7b70728eaf  Value=0
  Integrator +/- 50 deg/sec : Integrator  RequirementInfo={} %GIDa_184761dc_dd34_4e11_a9a1_45666f9633ce  InitialConditionSource=external  LimitOutput=on  UpperSaturationLimit=50  LowerSaturationLimit=-50
  ManualPitchScope : Scope  NumInputPorts=6
      settings: RequirementInfo={} %GIDa_72549fa5_a8e6_4d3b_bf81_fe2e4b3e3c78  YMin=-5~-5~-5~-5~-5~-5  YMax=5~5~5~5~5~5  SaveName=ScopeData8
  Multiport Switch : MultiPortSwitch  RequirementInfo={} %GIDa_0bbdf906_a541_496e_ad5f_ef6074c08306
  PS Gain deg/sec : Gain  RequirementInfo={} %GIDa_09e1b5ed_2df1_4c0f_904b_20e167337447  Gain=50
  "PS Shaping " : Fcn  RequirementInfo={} %GIDa_9891bdf4_4482_4f22_b04c_7f3b3c651217  Expr=u(1)*abs(u(1))^1.0
  PS deadband +/- 0.01 : DeadZone  RequirementInfo={} %GIDa_71456b35_56d8_498c_a711_662ff091bfe4  LowerValue=-0.01  UpperValue=0.01  SaturateOnIntegerOverflow=on
  PS limits +/- 1 : Saturate  RequirementInfo={} %GIDa_083f66c2_2dbf_45d3_b1f1_17b5236f221d  UpperLimit=1  LowerLimit=-1
  Pitchcmd : Subsystem  Tag=STV Subsys  RequirementInfo={} %GIDa_9c06165d_2ff1_49a5_beb3_607465ac55a7  LoadFcn=sigbuilder_block('load');  StartFcn=sigbuilder_block('start');  StopFcn=sigbuilder_block('stop');  ClipboardFcn=sigbuilder_block('clipboard');  mask(Sigbuilder block){}
      mask help: Sigbuilder GUI
      mask init:
      | if ~strcmp(get_param(bdroot(gcbh),'SimulationStatus'),'stopped') tuvar = sigbuilder_block('maskInit'); end
      settings: CopyFcn=sigbuilder_block('copy');  DeleteFcn=sigbuilder_block('delete');  ModelCloseFcn=sigbuilder_block('modelClose');  PreSaveFcn=sigbuilder_block('preSave');  PauseFcn=sigbuilder_block('pause')  ContinueFcn=sigbuilder_block('continue')  NameChangeFcn=sigbuilder_block('namechange');  OpenFcn=sigbuilder_block('open',[159.36 418.56 676.8 484.8 ]);  CloseFcn=sigbuilder_block('close');
      mask Display: plot(0,0,100,100,[10,10,40,40,10],[80,20,20,80,80],[40,10],[50,50], [40,27,10],[65,72,56],[40,25,25,10],[28,28,43,43]);
  PitchCmd : Outport  RequirementInfo={} %GIDa_190ac238_936a_4f44_a6cf_756574c6088e
  wires:
  Pitchcmd/2(Signal 2) -> Multiport Switch/4
  Pitchcmd/1(Signal 1) -> Multiport Switch/3
  Constant1/1 -> Multiport Switch/2
  Constant/1 -> Multiport Switch/1
  Multiport Switch/1 -> ManualPitchScope/1, PS limits +/- 1/1  "stick"
  Thetafiltdeg/1 -> Integrator +/- 50 deg/sec/2
  Integrator +/- 50 deg/sec/1 -> ManualPitchScope/6, PitchCmd/1  "pitchcmd"
  PS Gain deg/sec/1 -> ManualPitchScope/5, Integrator +/- 50 deg/sec/1  "q_cmd"
  PS deadband +/- 0.01/1 -> ManualPitchScope/3, "PS Shaping "/1  "stkdb"
  PS limits +/- 1/1 -> ManualPitchScope/2, PS deadband +/- 0.01/1  "stklim"
  "PS Shaping "/1 -> ManualPitchScope/4, PS Gain deg/sec/1  "stkshape"

== system TCM_controls/Controls/ManualRollcmd ==
  rollfiltdeg : Inport  RequirementInfo={} %GIDa_07a92dc5_ffb9_45ec_9cef_77b6a233d40f
  Constant1 : Constant  RequirementInfo={} %GIDa_611e9103_b682_467f_9c82_dbfa31f41929  Value=0
  Integrator +/- 225 deg/sec : Integrator  RequirementInfo={} %GIDa_e78617ab_7fab_4ba5_a898_3550360eca64  InitialConditionSource=external  LimitOutput=on  UpperSaturationLimit=225  LowerSaturationLimit=-225
  ManualRollScope : Scope  NumInputPorts=6
      settings: RequirementInfo={} %GIDa_5f63eb68_4da6_47ff_a509_81151c652b7d  YMin=-5~-5~-5~-5~-5~-5  YMax=5~5~5~5~5~5  SaveName=ScopeData9
  Multiport Switch : MultiPortSwitch  RequirementInfo={} %GIDa_5aea403f_734f_4752_89a0_71dca3a49ae9
  RS Gain deg/sec : Gain  RequirementInfo={} %GIDa_0ebb9c7b_de10_4fce_a883_7618fc80f743  Gain=225
  "RS Shaping " : Fcn  RequirementInfo={} %GIDa_ff67ecae_6f44_462d_8520_e73f3d40923c  Expr=u(1)*abs(u(1))^1.0
  RS deadband +/- 0.01 : DeadZone  RequirementInfo={} %GIDa_e23b64ba_f027_4f1c_9e1c_ba6225723fa3  LowerValue=-0.01  UpperValue=0.01  SaturateOnIntegerOverflow=on
  RS limits +/- 1 : Saturate  RequirementInfo={} %GIDa_aebca1d4_5907_4c32_a7a6_c4645243ee5d  UpperLimit=1  LowerLimit=-1
  Rollcmd : Subsystem  Tag=STV Subsys  RequirementInfo={} %GIDa_d7b0b3c0_4dde_4284_8b84_0e70602adc83  LoadFcn=sigbuilder_block('load');  StartFcn=sigbuilder_block('start');  StopFcn=sigbuilder_block('stop');  ClipboardFcn=sigbuilder_block('clipboard');  mask(Sigbuilder block){}
      mask help: Sigbuilder GUI
      mask init:
      | if ~strcmp(get_param(bdroot(gcbh),'SimulationStatus'),'stopped') tuvar = sigbuilder_block('maskInit'); end
      settings: CopyFcn=sigbuilder_block('copy');  DeleteFcn=sigbuilder_block('delete');  ModelCloseFcn=sigbuilder_block('modelClose');  PreSaveFcn=sigbuilder_block('preSave');  PauseFcn=sigbuilder_block('pause')  ContinueFcn=sigbuilder_block('continue')  NameChangeFcn=sigbuilder_block('namechange');  OpenFcn=sigbuilder_block('open',[159.36 418.56 676.8 484.8 ]);  CloseFcn=sigbuilder_block('close');
      mask Display: plot(0,0,100,100,[10,10,40,40,10],[80,20,20,80,80],[40,10],[50,50], [40,27,10],[65,72,56],[40,25,25,10],[28,28,43,43]);
  portselect : Constant  RequirementInfo={} %GIDa_9188e8a5_be00_4b0e_ba57_ab9b1636fd57
  RollCmd : Outport  RequirementInfo={} %GIDa_2b9aed7d_f7b2_47e9_aeaa_54bc5b5cb372
  wires:
  rollfiltdeg/1 -> Integrator +/- 225 deg/sec/2
  Rollcmd/2(Signal 2) -> Multiport Switch/4
  Rollcmd/1(Signal 1) -> Multiport Switch/3
  Constant1/1 -> Multiport Switch/2
  Multiport Switch/1 -> ManualRollScope/1, RS limits +/- 1/1  "rollstick"
  Integrator +/- 225 deg/sec/1 -> ManualRollScope/6, RollCmd/1  "rollcmd"
  RS Gain deg/sec/1 -> ManualRollScope/5, Integrator +/- 225 deg/sec/1  "p_cmd"
  RS deadband +/- 0.01/1 -> ManualRollScope/3, "RS Shaping "/1  "rstkdb"
  RS limits +/- 1/1 -> ManualRollScope/2, RS deadband +/- 0.01/1  "rstklim"
  "RS Shaping "/1 -> ManualRollScope/4, RS Gain deg/sec/1  "rstkshape"
  portselect/1 -> Multiport Switch/1

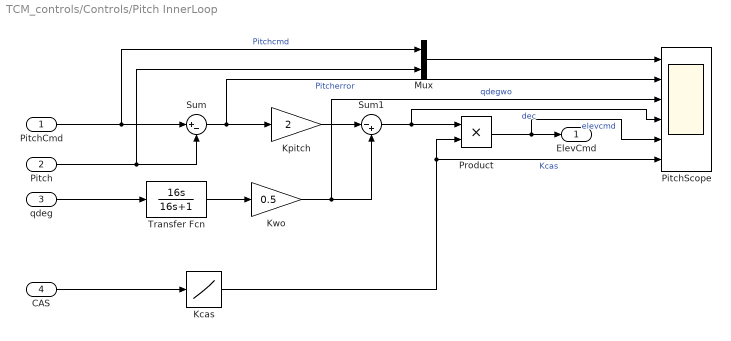
== system TCM_controls/Controls/Pitch InnerLoop ==
  PitchCmd : Inport  RequirementInfo={} %GIDa_4a5c3c54_da5b_4108_a300_efaa397132d5
  Pitch : Inport  RequirementInfo={} %GIDa_265949af_4cf8_438e_ace2_d11cfbdb00ea  Port=2
  qdeg : Inport  RequirementInfo={} %GIDa_b07e2a36_990b_4e65_a49a_64a6e3665fde  Port=3
  CAS : Inport  RequirementInfo={} %GIDa_66e3bdd2_8551_4394_ac28_f5b19f937929  Port=4
  Kcas : Lookup  RequirementInfo={} %GIDa_0965610f_1894_49ce_a11b_881a9dc869fa  InputValues=[0 120 350 500]  Table=[1.0 1.0 0.3 0.3]
  Kpitch : Gain  RequirementInfo={} %GIDa_65ab1a7f_3fa5_4118_886b_e9da348d80be  Gain=2
  Kwo : Gain  RequirementInfo={} %GIDa_51f608ef_523a_4f71_93de_8428d519d4eb  Gain=0.5
  Mux : Mux  RequirementInfo={} %GIDa_985ca14b_0594_42e3_afbf_19bd92eb9386  Inputs=2
  PitchScope : Scope  NumInputPorts=6
      settings: RequirementInfo={} %GIDa_e1f51da7_4b81_4006_8cc4_9d58d15037be  YMin=-2~-2~-2~-20~-20~0  YMax=10~2~2~20~20~1.2  SaveName=ScopeData11
  Product : Product  RequirementInfo={} %GIDa_dadaa5e8_c414_4af6_a28e_d782f4698e54  RndMeth=Zero
  Sum : Sum  RequirementInfo={} %GIDa_91d37d00_375f_4853_a756_2ba9297ebd49  Inputs=|+-
  Sum1 : Sum  RequirementInfo={} %GIDa_beb421ed_cee2_4789_8304_177a7de6f123  Inputs=|-+
  Transfer Fcn : TransferFcn  RequirementInfo={} %GIDa_1e358233_ad87_47bc_a348_d09b0b8a8e43  Numerator=[16 0]  Denominator=[16 1]
  ElevCmd : Outport  RequirementInfo={} %GIDa_01f368a7_325a_4dc3_b909_1ace73cb3a56
  wires:
  Sum/1 -> Kpitch/1, PitchScope/2  "Pitcherror"
  Pitch/1 -> Sum/2, Mux/2
  Kpitch/1 -> Sum1/1
  qdeg/1 -> Transfer Fcn/1
  Transfer Fcn/1 -> Kwo/1
  CAS/1 -> Kcas/1
  Sum1/1 -> Product/1, PitchScope/4  "dec"
  Kcas/1 -> Product/2, PitchScope/6  "Kcas"
  Product/1 -> ElevCmd/1, PitchScope/5  "elevcmd"
  Kwo/1 -> Sum1/2, PitchScope/3  "qdegwo"
  PitchCmd/1 -> Sum/1, Mux/1  "Pitchcmd"
  Mux/1 -> PitchScope/1

== system TCM_controls/Controls/PitchCmd ==
  Pitchcmd1 : Subsystem  Tag=STV Subsys  RequirementInfo={} %GIDa_7a3f0139_0acf_4d06_b83d_50aef399799b  LoadFcn=sigbuilder_block('load');  StartFcn=sigbuilder_block('start');  StopFcn=sigbuilder_block('stop');  ClipboardFcn=sigbuilder_block('clipboard');  mask(Sigbuilder block){}
      mask help: Sigbuilder GUI
      mask init:
      | if ~strcmp(get_param(bdroot(gcbh),'SimulationStatus'),'stopped') tuvar = sigbuilder_block('maskInit'); end
      settings: CopyFcn=sigbuilder_block('copy');  DeleteFcn=sigbuilder_block('delete');  ModelCloseFcn=sigbuilder_block('modelClose');  PreSaveFcn=sigbuilder_block('preSave');  PauseFcn=sigbuilder_block('pause')  ContinueFcn=sigbuilder_block('continue')  NameChangeFcn=sigbuilder_block('namechange');  OpenFcn=sigbuilder_block('open',[437.6 199.2 550.4 400 ]);  CloseFcn=sigbuilder_block('close');
      mask Display: plot(0,0,100,100,[10,10,40,40,10],[80,20,20,80,80],[40,10],[50,50], [40,27,10],[65,72,56],[40,25,25,10],[28,28,43,43]);
  Sum1 : Sum  RequirementInfo={} %GIDa_a4deae1d_5cfc_48e1_9bec_9c0390257841  Inputs=|++
  Trim Pitch : Constant  RequirementInfo={} %GIDa_dc863d23_1239_4418_b0db_bbac75085f61  Value=StatesInp(11)*180/pi
  Cmd : Outport  RequirementInfo={} %GIDa_8c80a7ec_2ff2_44b9_be1b_27dd3de93207
  wires:
  Pitchcmd1/1(Signal 1) -> Sum1/1
  Trim Pitch/1 -> Sum1/2
  Sum1/1 -> Cmd/1

== system TCM_controls/Controls/Roll InnerLoop ==
  note: orig =[0 60 140]
  note: orig = 0.25
  note: orig = 0.8
  RollCmd : Inport  RequirementInfo={} %GIDa_c4250928_4564_4cab_a5c8_d68e6317c8b4
  Roll : Inport  RequirementInfo={} %GIDa_9914bad1_a72d_4b74_9a98_1dcf7a16f2fd  Port=2
  pdeg : Inport  RequirementInfo={} %GIDa_07a05b66_3898_4974_ab1f_9227d6ab4e06  Port=3
  CAS : Inport  RequirementInfo={} %GIDa_1a4ab018_6653_4bbb_a5d2_4e34b83c521e  Port=4
  Kcas : Lookup  RequirementInfo={} %GIDa_896b12bd_69fe_41b2_8fe2_e545412da4b1  InputValues=[0 120 350 500]  Table=[1.0 1.0 0.3 0.3]
  Kphierr : Gain  RequirementInfo={} %GIDa_d760e33e_c337_4300_aa09_de760e2b7a59  Gain=0.5
  Product : Product  RequirementInfo={} %GIDa_759f9cd4_6466_4a5f_a26b_64825aaeb055  RndMeth=Zero
  Roll_IL_scope : Scope  NumInputPorts=7
      settings: RequirementInfo={} %GIDa_e41087de_1a00_450f_8337_aab8927c6c66  YMin=-30~-30~-10~-10~-4~-10~0  YMax=30~30~10~10~4~10~1  SaveName=ScopeData5
  Sum : Sum  RequirementInfo={} %GIDa_13272a0f_e3af_43ea_bc64_8a5c68520b41  Inputs=|+-
  Sum1 : Sum  RequirementInfo={} %GIDa_e1b8ada5_bac1_49bb_b3ab_dee833b4d259  Inputs=|+-
  rollrate_IL : ZeroPole  RequirementInfo={} %GIDa_86bfc316_824f_4222_9eb4_be2cdc9d443a  Zeros=0  Poles=-0.5  Gain=0.00645
  AilCmd : Outport  RequirementInfo={} %GIDa_6976c97e_4a9f_46e4_90da_05ce34dfac9b
  wires:
  Product/1 -> AilCmd/1, Roll_IL_scope/6  "ailcmd"
  Kcas/1 -> Product/2, Roll_IL_scope/7  "kcas"
  Sum1/1 -> Product/1
  CAS/1 -> Kcas/1
  rollrate_IL/1 -> Sum1/2, Roll_IL_scope/5  "pdegwo"
  pdeg/1 -> rollrate_IL/1, Roll_IL_scope/4  "pdeg"
  Kphierr/1 -> Sum1/1
  Roll/1 -> Sum/2, Roll_IL_scope/2  "roll"
  Sum/1 -> Kphierr/1, Roll_IL_scope/3  "rollerr"
  RollCmd/1 -> Sum/1, Roll_IL_scope/1  "rollcmd"
